simulink model "gol_mat_simulink_tb"  (R2021b)
settings: Solver=VariableStepAuto  StartTime=0.0  StopTime=1  RelTol=1e-3
values from neighbouring files (symbols this model uses):
  filter = [ ... (first row only)    [gol_mat_tb.m]
undefined symbols (not defined in the file or in its folder): columns, input_img
libraries: dspsrcs4 x1
settings Model: Creator=torha  LastModifiedBy=torha

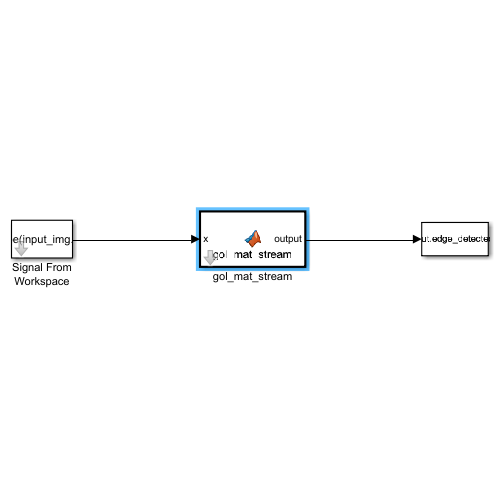
[thumbnail: Simulink's stored preview of the top-level diagram]
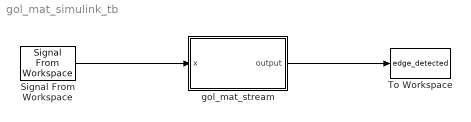
== system gol_mat_simulink_tb ==
  Signal From Workspace : dspsrcs4/Signal From Workspace  X=reshape(input_img.', 1, [])  Ts=1/length(input_img(:))  nsamps=1  OutputAfterFinalValue=Setting to zero  ignoreOrWarnInputAndFrameLengths=off  OutputFrames=off
  To Workspace : ToWorkspace  VariableName=edge_detected  SampleTime=-1
  gol_mat_stream : MATLAB Function  TreatAsAtomicUnit=on  mask{width=columns, kernel=filter}
  wires:
  Signal From Workspace/1 -> gol_mat_stream/1(x)
  gol_mat_stream/1(output) -> To Workspace/1

== matlab function gol_mat_simulink_tb/gol_mat_stream ==
  data: x input; output output; width parameter; kernel parameter
function output = gol_mat_stream(x, width, kernel)
    [kernel_height, kernel_width] = size(kernel);

    persistent memory;
    persistent extraMemory;
    if isempty(memory) || isempty(extraMemory)
        memory = zeros(kernel_height-1, width);
        extraMemory = zeros(1, kernel_width-1);
    end
    
    flipped_kernel = flip(flip(kernel,2));
    output = sum([x, extraMemory].*flipped_kernel(1,:));

    for i=1:kernel_height-1
        output = output + sum(memory(i, end-kernel_width+1:end).*flipped_kernel(i+1,:));
    end
    
    memory = [
        extraMemory(end), memory(1, 1:end-1);
        memory(1:end-1,end), memory(2:end,1:end-1);
    ];

    extraMemory = [x, extraMemory(1:end-1)];

end
